simulink model "UAV_Fleet2"  (R2013b)
settings: Solver=ode1  StartTime=0.0  StopTime=300  FixedStep=simPars.SampleTime  RelTol=1e-3
undefined symbols (not defined in the file or in its folder): AC_Fleet, DiscIntNeverNeededParam, Earth, Env, eul_0, m, s, simPars, WGS84
libraries: simulink x23, Actuator_Lib x5, aerolib6dofsys x4, aerolibasang x3, instrumentlib x2, aerolibconvert2 x2, aerolibtransform2 x2, etargetslib x1, aerolibutil x1, aerolibatmos2 x1, aerolibobsolete x1, aerolibgravity2 x1
(part 1 of 2)
settings Model: Creator=Paul Freeman  LastModifiedBy=descobar
settings DataIOCC: LimitDataPoints=off  SignalLoggingSaveFormat=ModelDataLogs  SaveOutput=off  SignalLogging=off
settings OptimizationCC: ExpressionDepthLimit=2147483647
settings DebuggingCC: FcnCallInpInsideContextMsg=UseLocalSettings  StateNameClashWarn=warning
settings HardwareCC: ProdLargestAtomicInteger=Long  ProdLargestAtomicFloat=Double  ProdIntDivRoundTo=Zero  ProdEndianess=BigEndian  ProdHWDeviceType=Freescale->32-bit PowerPC
settings SFSimCC: SimParseCustomCode=off
settings GRTTargetCC: CombineOutputUpdateFcns=off  GRTInterface=on

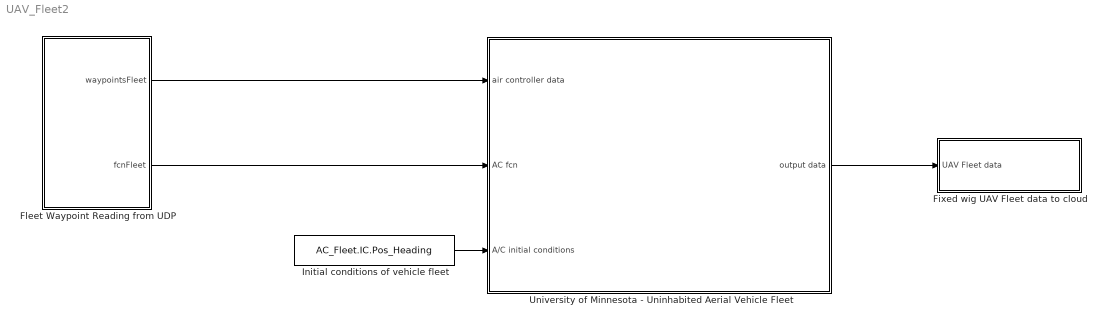
== system UAV_Fleet2 ==
  Fixed wig UAV Fleet data to cloud : Subsystem
  Fleet Waypoint Reading from UDP : Subsystem
  Initial conditions of vehicle fleet : Constant  Value=AC_Fleet.IC.Pos_Heading  VectorParams1D=off
  University of Minnesota - Uninhabited Aerial Vehicle Fleet : Subsystem  TreatAsAtomicUnit=on  mask{AC=AC_Fleet.AC, Env=Env, SampleTime=simPars.SampleTime}
      mask prompts: AC "Aircraft properties"; Env "Environmental parameters"; SampleTime "Sample time (sec)"
  wires:
  Initial conditions of vehicle fleet/1 -> University of Minnesota - Uninhabited Aerial Vehicle Fleet/3(A/C initial conditions)
  University of Minnesota - Uninhabited Aerial Vehicle Fleet/1(output data) -> Fixed wig UAV Fleet data to cloud/1(UAV Fleet data)
  Fleet Waypoint Reading from UDP/1(waypointsFleet) -> University of Minnesota - Uninhabited Aerial Vehicle Fleet/1(air controller data)
  Fleet Waypoint Reading from UDP/2(fcnFleet) -> University of Minnesota - Uninhabited Aerial Vehicle Fleet/2(AC fcn)

== system UAV_Fleet2/Fixed wig UAV Fleet data to cloud ==
  UAV Fleet data : Inport
  Rate Transition : RateTransition  OutPortSampleTime=simPars.SampleTime*5
  UDP Send : instrumentlib/UDP Send  Host=localhost  Port=9090  LocalPort=9091  EnableBlockingMode=on  ByteOrder=BigEndian
  wires:
  Rate Transition/1 -> UDP Send/1
  UAV Fleet data/1 -> Rate Transition/1

== system UAV_Fleet2/Fleet Waypoint Reading from UDP ==
  Byte Unpack : etargetslib/Byte Unpack  dimensions={[3],[2],[30], [1]}  datatypes={'uint8', 'uint16', 'double','uint16'}  byteAlign=1
  "DataBase " : MATLAB Function  TreatAsAtomicUnit=on
  Demux1 : Demux  Outputs=2
  UDP Receive : instrumentlib/UDP Receive  Host=localhost  Port=9040  LocalPort=9040  DataSize="[249    1]"  EnableBlockingMode=off  Timeout=10  SampleTime=0.02  DataType=uint8  ByteOrder=BigEndian
  term0 : Terminator
  term1 : Terminator
  waypointsFleet : Outport
  fcnFleet : Outport  Port=2
  wires:
  "DataBase "/1(dataFleet) -> waypointsFleet/1
  Demux1/2 -> "DataBase "/2(functionID)
  UDP Receive/2 -> "DataBase "/4(status)
  Demux1/1 -> "DataBase "/1(uavID)
  Byte Unpack/3 -> "DataBase "/3(dataUAV)
  Byte Unpack/2 -> Demux1/1
  UDP Receive/1 -> Byte Unpack/1
  "DataBase "/2(fcnFleet) -> fcnFleet/1
  Byte Unpack/1 -> term0/1
  Byte Unpack/4 -> term1/1

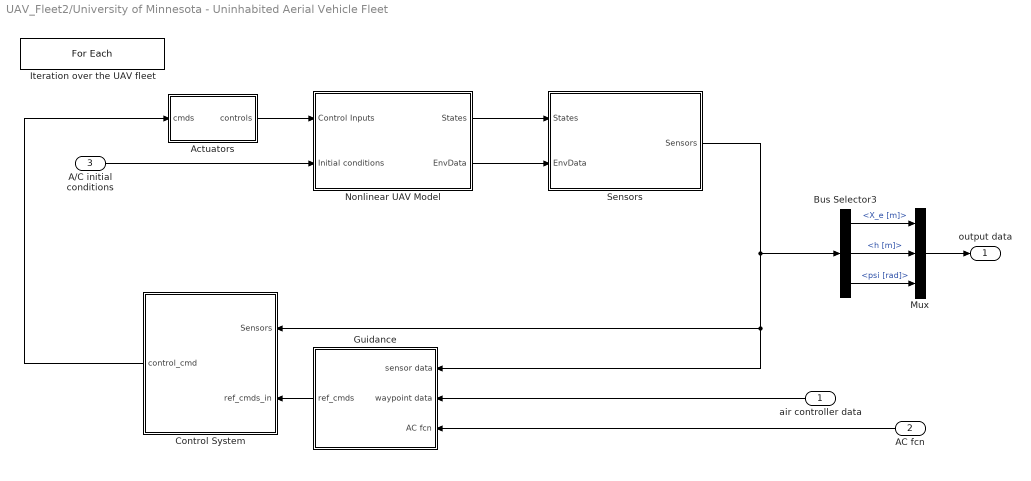
== system UAV_Fleet2/University of Minnesota - Uninhabited Aerial Vehicle Fleet ==
  air controller data : Inport  Partition=on  PartitionDimension=3  PartitionWidth=1
  AC fcn : Inport  Port=2  Partition=on  PartitionDimension=1  PartitionWidth=1
  A/C initial conditions : Inport  Port=3  Partition=on  PartitionDimension=2  PartitionWidth=1
  Actuators : Subsystem
  Bus Selector3 : BusSelector  OutputSignals=X_e [m],h [m],psi [rad]
  Control System : Subsystem  mask{control=AC.FC.control, IntegerTimeDelay=AC.FC.IntegerTimeDelay, TrimCondition=AC.TrimCondition, OperatingPoint=AC.OperatingPoint}
      mask prompts: control "Controller parameters"; IntegerTimeDelay "Integer Time Delay"; TrimCondition "Trim Condition"; OperatingPoint "Operating Point"
  "Guidance " : Subsystem
  Iteration over the UAV fleet : ForEach  DisableCoverage=on  IndexMode=One-based
  Mux : Mux  Inputs=3
  Nonlinear UAV Model : Subsystem  mask{TrimCondition=AC.TrimCondition}
      mask prompts: TrimCondition "Trim Condition"
  Sensors : Subsystem
  output data : Outport  ConcatenationDimension=1
  wires:
  Sensors/1(Sensors) -> "Guidance "/1(sensor data), Control System/1(Sensors), Bus Selector3/1
  Nonlinear UAV Model/1(States) -> Sensors/1(States)
  Nonlinear UAV Model/2(EnvData) -> Sensors/2(EnvData)
  Control System/1(control_cmd) -> Actuators/1(cmds)
  Actuators/1(controls) -> Nonlinear UAV Model/1(Control Inputs)
  "Guidance "/1(ref_cmds) -> Control System/2(ref_cmds_in)
  air controller data/1 -> "Guidance "/2(waypoint data)
  A/C initial conditions/1 -> Nonlinear UAV Model/2(Initial conditions)
  Bus Selector3/1 -> Mux/1  "<X_e [m]>"
  Bus Selector3/2 -> Mux/2  "<h [m]>"
  Mux/1 -> output data/1
  Bus Selector3/3 -> Mux/3  "<psi [rad]>"
  AC fcn/1 -> "Guidance "/3(AC fcn)

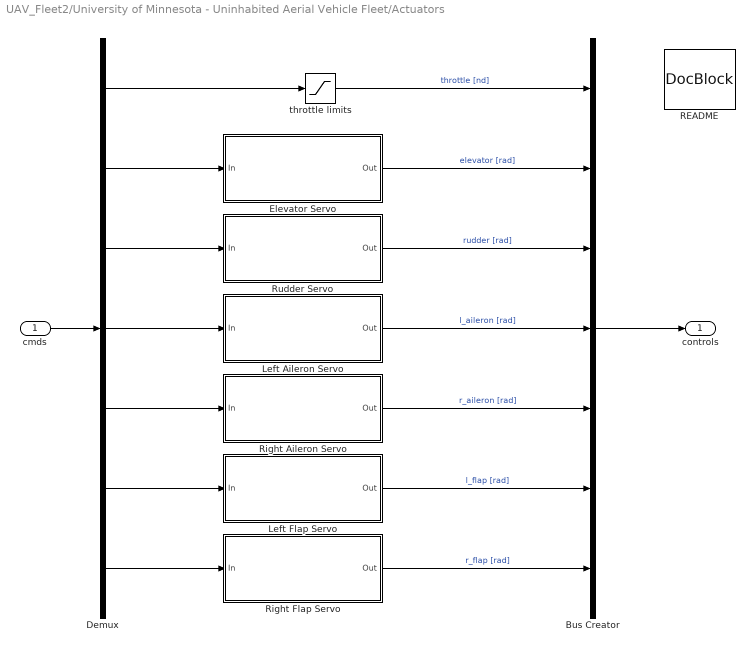
== system UAV_Fleet2/University of Minnesota - Uninhabited Aerial Vehicle Fleet/Actuators ==
  cmds : Inport
  Bus Creator : BusCreator  Inputs=7
  Demux : Demux  Outputs=7
  Elevator Servo : Subsystem  mask(Rate and Position Limited Servo){freq=AC.Actuator.elevator.BW, RL=AC.Actuator.elevator.RateLim, POS_hi=AC.Actuator.elevator.PosLim, POS_lo=AC.Actuator.elevator.NegLim}
      mask prompts: freq "Bandwidth, Hz"; RL "Rate Limit:"; POS_hi "Position Limit High:"; POS_lo "Position Limit Low:"
      mask help: First order transfer function: w/(s+w), with rate and position limits.
      mask Help:
      | This block models a first order servo with the initial condition
      | on the integrator set to the steady state value for constant input.
      | The servo is rate and position limited and those values are set
      | in the block parameters.
      mask Display:
      | text(.48,.55,sprintf('%3.1f Hz\nBW',freq),'horizontalAlignment','center');
      | 
      | text(0.18,0.45,sprintf('|d/dt|\n<%0.1f',RL),'horizontalAlignment','center');
      | 
      | text(0.88,0.85,num2str(POS_hi),'horizontalAlignment', 'center');
      | text(0.88,0.2,num2str(POS_lo),'horizontalAlignment', 'center');
      | text(0.73,0.5,'P\nL');
      | 
      | 
      | plot([0.83 0.87 0.93 0.97],[0.4 0.4 0.6 0.6]);
      | plot([0.81 0.99],[0.5 0.5]);
      | plot([0.9 0.9],[0.3 0.7]);
      | plot([0.81 0.99 0.99 0.81 0.81],[0.3 0.3 0.7 0.7 0.3]);
  Left Aileron Servo : Subsystem  mask(Rate and Position Limited Servo){freq=AC.Actuator.l_aileron.BW, RL=AC.Actuator.l_aileron.RateLim, POS_hi=AC.Actuator.l_aileron.PosLim, POS_lo=AC.Actuator.l_aileron.NegLim}
      mask prompts: freq "Bandwidth, Hz"; RL "Rate Limit:"; POS_hi "Position Limit High:"; POS_lo "Position Limit Low:"
      mask help: First order transfer function: w/(s+w), with rate and position limits.
      mask Help:
      | This block models a first order servo with the initial condition
      | on the integrator set to the steady state value for constant input.
      | The servo is rate and position limited and those values are set
      | in the block parameters.
      mask Display:
      | text(.48,.55,sprintf('%3.1f Hz\nBW',freq),'horizontalAlignment','center');
      | 
      | text(0.18,0.45,sprintf('|d/dt|\n<%0.1f',RL),'horizontalAlignment','center');
      | 
      | text(0.88,0.85,num2str(POS_hi),'horizontalAlignment', 'center');
      | text(0.88,0.2,num2str(POS_lo),'horizontalAlignment', 'center');
      | text(0.73,0.5,'P\nL');
      | 
      | 
      | plot([0.83 0.87 0.93 0.97],[0.4 0.4 0.6 0.6]);
      | plot([0.81 0.99],[0.5 0.5]);
      | plot([0.9 0.9],[0.3 0.7]);
      | plot([0.81 0.99 0.99 0.81 0.81],[0.3 0.3 0.7 0.7 0.3]);
  Left Flap Servo : Subsystem  mask(Rate and Position Limited Servo){freq=AC.Actuator.l_flap.BW, RL=AC.Actuator.l_flap.RateLim, POS_hi=AC.Actuator.l_flap.PosLim, POS_lo=AC.Actuator.l_flap.NegLim}
      mask prompts: freq "Bandwidth, Hz"; RL "Rate Limit:"; POS_hi "Position Limit High:"; POS_lo "Position Limit Low:"
      mask help: First order transfer function: w/(s+w), with rate and position limits.
      mask Help:
      | This block models a first order servo with the initial condition
      | on the integrator set to the steady state value for constant input.
      | The servo is rate and position limited and those values are set
      | in the block parameters.
      mask Display:
      | text(.48,.55,sprintf('%3.1f Hz\nBW',freq),'horizontalAlignment','center');
      | 
      | text(0.18,0.45,sprintf('|d/dt|\n<%0.1f',RL),'horizontalAlignment','center');
      | 
      | text(0.88,0.85,num2str(POS_hi),'horizontalAlignment', 'center');
      | text(0.88,0.2,num2str(POS_lo),'horizontalAlignment', 'center');
      | text(0.73,0.5,'P\nL');
      | 
      | 
      | plot([0.83 0.87 0.93 0.97],[0.4 0.4 0.6 0.6]);
      | plot([0.81 0.99],[0.5 0.5]);
      | plot([0.9 0.9],[0.3 0.7]);
      | plot([0.81 0.99 0.99 0.81 0.81],[0.3 0.3 0.7 0.7 0.3]);
  README : simulink/Model-Wide Utilities/DocBlock  DocumentType=Text
      content=|
      | Actuators
      |
      | This block implements first order, rate and position limited actuator
      | models for the aileron, elevator, rudder and flap channels. The throttle
      | does not have a servo, but is position limited.
      |
      | Parameters for these models are contained in the aircraft configuration
      | data structure variable, "AC". Specfically,
      |
      | >> AC.Actuator
      |
      | ans =
      |
      |      elevator: [1x1 struct]
      |     l_aileron: [1x1 struct]
      |     r_aileron: [1x1 struct]
      |        rudder: [1x1 struct]
      |        l_flap: [1x1 struct]
      |        r_flap: [1x1 struct]
      |      throttle: [1x1 struct]
      |
      | Control Inputs Sign Convention
      | Elevator: +TED
      | Rudder: +TEL
      | Ailerons: +TED, da = (da_R-da_L)/2
      | Flaps: +TED
      | Throttle: always positive
  Right Aileron Servo : Subsystem  mask(Rate and Position Limited Servo){freq=AC.Actuator.r_aileron.BW, RL=AC.Actuator.r_aileron.RateLim, POS_hi=AC.Actuator.r_aileron.PosLim, POS_lo=AC.Actuator.r_aileron.NegLim}
      mask prompts: freq "Bandwidth, Hz"; RL "Rate Limit:"; POS_hi "Position Limit High:"; POS_lo "Position Limit Low:"
      mask help: First order transfer function: w/(s+w), with rate and position limits.
      mask Help:
      | This block models a first order servo with the initial condition
      | on the integrator set to the steady state value for constant input.
      | The servo is rate and position limited and those values are set
      | in the block parameters.
      mask Display:
      | text(.48,.55,sprintf('%3.1f Hz\nBW',freq),'horizontalAlignment','center');
      | 
      | text(0.18,0.45,sprintf('|d/dt|\n<%0.1f',RL),'horizontalAlignment','center');
      | 
      | text(0.88,0.85,num2str(POS_hi),'horizontalAlignment', 'center');
      | text(0.88,0.2,num2str(POS_lo),'horizontalAlignment', 'center');
      | text(0.73,0.5,'P\nL');
      | 
      | 
      | plot([0.83 0.87 0.93 0.97],[0.4 0.4 0.6 0.6]);
      | plot([0.81 0.99],[0.5 0.5]);
      | plot([0.9 0.9],[0.3 0.7]);
      | plot([0.81 0.99 0.99 0.81 0.81],[0.3 0.3 0.7 0.7 0.3]);
  Right Flap Servo : Subsystem  mask(Rate and Position Limited Servo){freq=AC.Actuator.l_flap.BW, RL=AC.Actuator.l_flap.RateLim, POS_hi=AC.Actuator.l_flap.PosLim, POS_lo=AC.Actuator.l_flap.NegLim}
      mask prompts: freq "Bandwidth, Hz"; RL "Rate Limit:"; POS_hi "Position Limit High:"; POS_lo "Position Limit Low:"
      mask help: First order transfer function: w/(s+w), with rate and position limits.
      mask Help:
      | This block models a first order servo with the initial condition
      | on the integrator set to the steady state value for constant input.
      | The servo is rate and position limited and those values are set
      | in the block parameters.
      mask Display:
      | text(.48,.55,sprintf('%3.1f Hz\nBW',freq),'horizontalAlignment','center');
      | 
      | text(0.18,0.45,sprintf('|d/dt|\n<%0.1f',RL),'horizontalAlignment','center');
      | 
      | text(0.88,0.85,num2str(POS_hi),'horizontalAlignment', 'center');
      | text(0.88,0.2,num2str(POS_lo),'horizontalAlignment', 'center');
      | text(0.73,0.5,'P\nL');
      | 
      | 
      | plot([0.83 0.87 0.93 0.97],[0.4 0.4 0.6 0.6]);
      | plot([0.81 0.99],[0.5 0.5]);
      | plot([0.9 0.9],[0.3 0.7]);
      | plot([0.81 0.99 0.99 0.81 0.81],[0.3 0.3 0.7 0.7 0.3]);
  Rudder Servo : Subsystem  mask(Rate and Position Limited Servo){freq=AC.Actuator.rudder.BW, RL=AC.Actuator.rudder.RateLim, POS_hi=AC.Actuator.rudder.PosLim, POS_lo=AC.Actuator.rudder.NegLim}
      mask prompts: freq "Bandwidth, Hz"; RL "Rate Limit:"; POS_hi "Position Limit High:"; POS_lo "Position Limit Low:"
      mask help: First order transfer function: w/(s+w), with rate and position limits.
      mask Help:
      | This block models a first order servo with the initial condition
      | on the integrator set to the steady state value for constant input.
      | The servo is rate and position limited and those values are set
      | in the block parameters.
      mask Display:
      | text(.48,.55,sprintf('%3.1f Hz\nBW',freq),'horizontalAlignment','center');
      | 
      | text(0.18,0.45,sprintf('|d/dt|\n<%0.1f',RL),'horizontalAlignment','center');
      | 
      | text(0.88,0.85,num2str(POS_hi),'horizontalAlignment', 'center');
      | text(0.88,0.2,num2str(POS_lo),'horizontalAlignment', 'center');
      | text(0.73,0.5,'P\nL');
      | 
      | 
      | plot([0.83 0.87 0.93 0.97],[0.4 0.4 0.6 0.6]);
      | plot([0.81 0.99],[0.5 0.5]);
      | plot([0.9 0.9],[0.3 0.7]);
      | plot([0.81 0.99 0.99 0.81 0.81],[0.3 0.3 0.7 0.7 0.3]);
  throttle limits : Saturate  UpperLimit=AC.Actuator.throttle.PosLim  LowerLimit=AC.Actuator.throttle.NegLim
  controls : Outport
  wires:
  Bus Creator/1 -> controls/1
  cmds/1 -> Demux/1
  Demux/1 -> throttle limits/1
  throttle limits/1 -> Bus Creator/1  "throttle [nd]"
  Demux/2 -> Elevator Servo/1(In)
  Elevator Servo/1(Out) -> Bus Creator/2  "elevator [rad]"
  Demux/3 -> Rudder Servo/1(In)
  Rudder Servo/1(Out) -> Bus Creator/3  "rudder [rad]"
  Demux/4 -> Left Aileron Servo/1(In)
  Left Aileron Servo/1(Out) -> Bus Creator/4  "l_aileron [rad]"
  Demux/6 -> Left Flap Servo/1(In)
  Left Flap Servo/1(Out) -> Bus Creator/6  "l_flap [rad]"
  Right Aileron Servo/1(Out) -> Bus Creator/5  "r_aileron [rad]"
  Right Flap Servo/1(Out) -> Bus Creator/7  "r_flap [rad]"
  Demux/7 -> Right Flap Servo/1(In)
  Demux/5 -> Right Aileron Servo/1(In)

== system UAV_Fleet2/University of Minnesota - Uninhabited Aerial Vehicle Fleet/Control System ==
  note: See "Software\Documentation\UAV_controllaw_ICD.pdf" for
      | details on the input/output signals.
  Sensors : Inport
  ref_cmds_in : Inport  Port=2
  Bus Creator : BusCreator  Inputs=7
  Bus Selector1 : BusSelector  OutputSignals=phi [rad],theta [rad],psi [rad],p [rad/s],q [rad/s],r [rad/s],Ax [m/s^2],Ay [m/s^2],Az [m/s^2],h [m],V_s [m/s],alpha [rad],beta [rad],Geodetic Latitude [rad],Geodetic Longitude [rad],Altitude [m],Xdot [m/s],Ydot [m/s],Zdot [m/s]  OutputAsBus=on
  "Control_Algorithm " : Subsystem
  Demux : Demux  Outputs=7
  Integer Delay : Delay  DelayLength=IntegerTimeDelay  InitialCondition=repmat([TrimCondition.AttitudeIni;TrimCondition.RatesIni;TrimCondition.AccelsIni;OperatingPoint.op_report.Outputs(4).y;TrimCondition.WindAxesIni;TrimCondition.LLIni;0; zeros(3,1)],[1,IntegerTimeDelay])  InputProcessing=Inherited
  README : simulink/Model-Wide Utilities/DocBlock  DocumentType=Text
      content=|
      | Control Law Block
      |
      | This block uses Model Referencing to allow the user to easily switch out
      | control law implementations. An example usage would be first a user develops
      | a control law using simulink blocks. This controller is referred to as the
      | "simulink controller" and would be selected by setting the variable
      | "controller_mode" to 2. Once the development is completed, the user then
      | implements the Simulink controller into C-code suitable for integration
      | with the UAV software. This controller is referred to as the "flight code"
      | and would be selected by setting "controller_mode" to 1.
      |
      | This is done using the Simulink.Variant object. See the documentation for
      | more detail. The user can specify any number of variants for the Control
      | Software block; edit the ModelReferenceParameters by right-clicking this
      | block to set which Simulink model is reference for each Variant object.
      | Note that these objects must be present in the base workspace. It
      | is strongly recommended that you use the "simulink_controller.mdl" file as
      | a starting place and "Save As" to a different file name.
      |
      | In summary, to switch the Control Software, modify the "contoller_mode"
      | variable:
      | 1 = flight code controller (C implementation)
      | 2 = simulink controller (empty simulink model)
      |
      |
      | See "Software\Documentation\UAV_controllaw_ICD.pdf" for details on the
      | input/output signals.
      |
      | The control_cmd signal must have the following order:
      | throttle
      | elevator
      | rudder
      | l_aileron
      | r_aileron
      | l_flap
      | r_flap
      |
      | Control Inputs Sign Convention
      | TED = Trailing Edge Down
      | TEL = Trailing Edge Left
      | ------------------------
      | Elevator: +TED
      | Rudder: +TEL
      | Aileron: +TED, da = (da_R-da_L)/2
      | Throttle: always positive
      | Flap: +TED
      |
      |
      | The refrence command signal must have the following order:
      | 1. phi_cmd
      | 2. theta_cmd
      | 3. psi_cmd
      | 4. p_cmd
      | 5. q_cmd
      | 6. r_cmd
      | 7. V_s_cmd
      | 8. h_cmd
      | 9. gndtrk_cmd
      | 10. aoa_cmd
      | 11. aos_cmd
      | 12. gamma_cmd
      | Note the trimmed value of pitch angle theta is included in the reference
      | command. Use the Doublet Generator block (or other signal generating block)
      | to input reference commands to the Control Software.
  Terminator : Terminator
  "Trim setting " : Actuator_Lib/Trim setting 
  control_cmd : Outport
  wires:
  "Control_Algorithm "/1(control_cmd1) -> "Trim setting "/1
  Sensors/1 -> Bus Selector1/1
  ref_cmds_in/1 -> "Control_Algorithm "/2(ref_cmds)
  Bus Creator/1 -> control_cmd/1
  Demux/1 -> Bus Creator/1  "throttle [nd]"
  Demux/2 -> Bus Creator/2  "elevator [rad]"
  Demux/3 -> Bus Creator/3  "rudder [rad]"
  Demux/4 -> Bus Creator/4  "l_aileron [rad]"
  Demux/5 -> Bus Creator/5  "r_aileron [rad]"
  Demux/6 -> Bus Creator/6  "l_flap [rad]"
  Demux/7 -> Bus Creator/7  "r_flap [rad]"
  Integer Delay/1 -> "Control_Algorithm "/1(feedback)
  Bus Selector1/1 -> Integer Delay/1
  "Trim setting "/1 -> Demux/1
  "Control_Algorithm "/2(ref_cmds_out) -> Terminator/1

== system UAV_Fleet2/University of Minnesota - Uninhabited Aerial Vehicle Fleet/Guidance  ==
  note: See /Software/Documentation/UAV_controlaw_ICD.pdf
      | for details
  sensor data : Inport
  waypoint data : Inport  Port=2
  AC fcn : Inport  Port=3
  Bus Selector1 : BusSelector  OutputSignals=psi [rad]
  Bus Selector2 : BusSelector  OutputSignals=X_e [m].X [m],X_e [m].Y [m],X_e [m].Z [m]
  Constant : Constant  Value=0
  Ground track angle computation based on waypoints : MATLAB Function  TreatAsAtomicUnit=on
  Model Info : simulink/Model-Wide Utilities/Model Info  InitialBlockCM=None  Frame=on  DisplayStringWithTags=|  HorizontalTextAlignment=Center  LeftAlignmentValue=0.5  SourceBlockDiagram=UAV_Fleet2  TagMaxNumber=20
      | Ref Cmd Port Info
      | 
      | 1. phi_cmd
      | 2. theta_cmd
      | 3. psi_cmd
      | 4. p_cmd
      | 5. q_cmd
      | 6. r_cmd
      | 7. V_s_cmd
      | 8. h_cmd
      | 9. gndtrk_cmd
      | 10. aoa_cmd
      | 11. aos_cmd
      | 12. gamma_cmd
  Mux : Mux  Inputs=12
  Mux1 : Mux  Inputs=3
  ref_cmds : Outport
  wires:
  Mux/1 -> ref_cmds/1
  Bus Selector2/1 -> Mux1/1  "<X [m]>"
  Bus Selector2/2 -> Mux1/2  "<Y [m]>"
  Bus Selector2/3 -> Mux1/3  "<Z [m]>"
  sensor data/1 -> Bus Selector1/1, Bus Selector2/1
  Bus Selector1/1 -> Ground track angle computation based on waypoints/2(psi)  "<psi [rad]>"
  Mux1/1 -> Ground track angle computation based on waypoints/3(Pned)
  waypoint data/1 -> Ground track angle computation based on waypoints/1(waypoint)
  Ground track angle computation based on waypoints/2(psiTarget) -> Mux/9
  Constant/1 -> Mux/3, Mux/4, Mux/5, Mux/6, Mux/7, Mux/10, Mux/11, Mux/12, Mux/1, Mux/2
  Ground track angle computation based on waypoints/1(hCmd) -> Mux/8
  AC fcn/1 -> Ground track angle computation based on waypoints/4(fcn)

== system UAV_Fleet2/University of Minnesota - Uninhabited Aerial Vehicle Fleet/Nonlinear UAV Model ==
  Control Inputs : Inport
  Initial conditions : Inport  Port=2
  6DoF EOM : Subsystem  mask(6DoF EoM (Body Axis)){units=Metric (MKS), mtype=Fixed, rep=Euler Angles, xme_0=TrimCondition.InertialIni, Vm_0=TrimCondition.VelocitiesIni, pm_0=TrimCondition.RatesIni, mass_0=AC.Mass, mass_e=0.5, mass_f=2.0, inertia=AC.Inertia.Matrix, inertia_e=eye(3), inertia_f=2*eye(3), k_quat=1.0}
      mask prompts: mtype "Mass type:"; rep "Representation:"; xme_0 "Initial position in inertial axes [Xe,Ye,Ze]:"; Vm_0 "Initial velocity in body axes [U,v,w]:"; pm_0 "Initial body rotation rates [p,q,r]:"; mass_0 "Initial mass:"; mass_e "Empty mass:"; mass_f "Full mass:"; inertia_e "Empty inertia matrix:"; inertia_f "Full inertia matrix:"; k_quat "Gain for quaternion normalization:"
      mask help:
      | Integrate the six-degrees-of-freedom equations of motion in body axis.
      |
      | This block has been modified from the original Aerospace Blockset
      | implementation. The inertial position vector (Xe) is no longer computed.
      | The original block did not have a way to add steady state winds to the
      | inertial velocities (Ve) prior to integrating to get Xe. Therefore, this
      | step is performed in the Auxiliary Equations block.
      mask Help: eval('asbhelp(''sixdof_euler_angles'')');
      mask TypeOptions units: Metric (MKS) | English (Velocity in ft/s) | English (Velocity in kts)
      mask TypeOptions mtype: Fixed | Simple Variable | Custom Variable
      mask Callback mtype: aeroicon('aeroblk6dofbody');
      mask TypeOptions rep: Euler Angles | Quaternion
      mask Callback rep: aeroicon('aeroblk6dofbody');
  Auxiliary Equations : Subsystem
  Environment : Subsystem
  Forces and Moments : Subsystem
  Initial conditions1 : InportShadow  Port=2
  "Packaging initial Euler angles " : Subsystem
  README : simulink/Model-Wide Utilities/DocBlock  DocumentType=Text
      content=|
      | Nonlinear UAV Model
      |
      | This block implements the nonlinear UAV dynamics model. Beginning on the
      | left, the Forces and Moments block models all of the relevant external
      | forces and moments acting on the aircraft.
      |
      | The 6DoF EOM block implements the six degree of freedom, fixed mass,
      | flat, non-rotating Earth, rigid body equations of motion. This block has
      | been modified from the original Aerospace Blockset implementation. The
      | inertial position vector (Xe) is no longer computed. The original block
      | did not have a way to add steady state winds to the inertial velocities
      | (Ve) prior to integrating to get Xe. Therefore, this step is performed in
      | the Auxiliary Equations block.
      |
      | The Auxiliary Equations computes other relevant variables (such as angle
      | of attack, indicated airspeed, etc) from state data. In this block are
      | the Navigation equations.
      |
      | Finally, the Environment block has Aerospace Blockset models for Earth's
      | atmosphere, gravity, and magnetic fields. Winds are modeled in two
      | portions: steady and unsteady. The steady portion is defined by a speed
      | and direction, and is horizontal only. The unsteady portion is made up of
      | a wind shear model and a turbulence model.
  States : Outport
  EnvData : Outport  Port=2
  wires:
  6DoF EOM/6(Ab) -> Auxiliary Equations/6(A_b)
  6DoF EOM/5(pdot,qdot,rdot) -> Auxiliary Equations/5(AngAccel)
  6DoF EOM/4(p,q,r) -> Auxiliary Equations/4(AngVel)
  6DoF EOM/3(Vb) -> Auxiliary Equations/3(V_b)
  6DoF EOM/2(DCM) -> Auxiliary Equations/2(DCM)
  6DoF EOM/1(Euler) -> Auxiliary Equations/1(Euler)
  Control Inputs/1 -> Forces and Moments/1(Control Inputs)
  Forces and Moments/1(Total Force) -> 6DoF EOM/1(Forces)
  Forces and Moments/2(Total Moment) -> 6DoF EOM/2(Moments)
  Auxiliary Equations/1(States) -> States/1, Forces and Moments/2(States), Environment/1(States)
  Forces and Moments/3(nonGravForces) -> Auxiliary Equations/7(NonGravForces)
  Environment/1(EnvData) -> Forces and Moments/3(EnvData), Auxiliary Equations/8(EnvData), EnvData/1
  Initial conditions/1 -> Auxiliary Equations/9(Initial conditions)
  Initial conditions1/1 -> "Packaging initial Euler angles "/1(Position and heading)
  "Packaging initial Euler angles "/1(Initial Euler angles) -> 6DoF EOM/3(Euler ini. (rad))

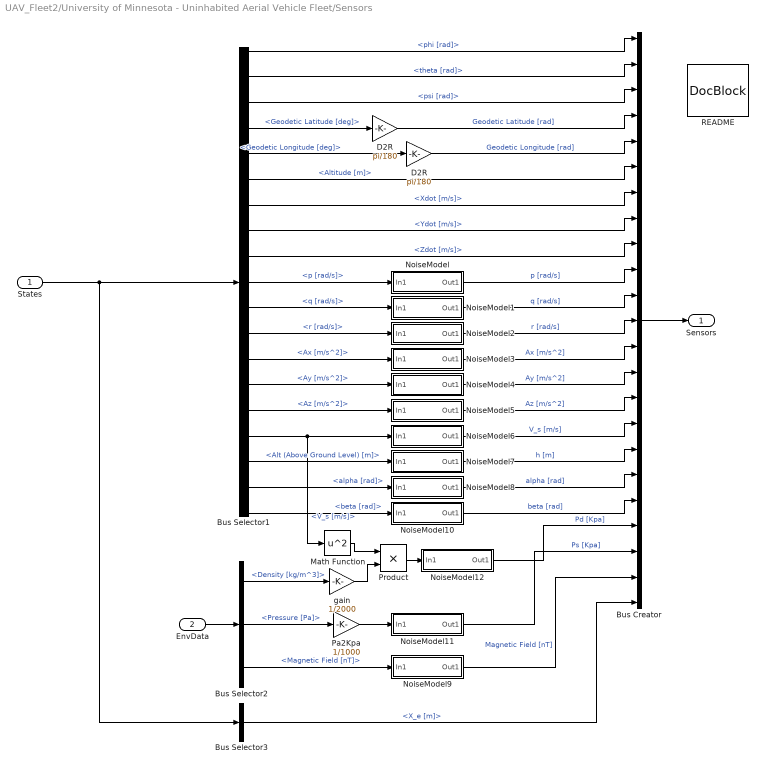
== system UAV_Fleet2/University of Minnesota - Uninhabited Aerial Vehicle Fleet/Sensors ==
  States : Inport
  EnvData : Inport  Port=2
  Bus Creator : BusCreator  Inputs=23
  Bus Selector1 : BusSelector  OutputSignals=Euler [rad].phi [rad],Euler [rad].theta [rad],Euler [rad].psi [rad],Nav.Geodetic Latitude [deg],Nav.Geodetic Longitude [deg],Nav.Altitude [m],V_e [m/s].Xdot [m/s],V_e [m/s].Ydot [m/s],V_e [m/s].Zdot [m/s],AngVel [rad/s].p [rad/s],AngVel [rad/s].q [rad/s],AngVel [rad/s].r [rad/s],Accels [m/s^2].Ax [m/s^2],Accels [m/s^2].Ay [m/s^2],Accels [m/s^2].Az [m/s^2],WindAxesParam.V_s [m/s],Nav.Alt (Above Ground Level) [m],WindAxesParam.alpha [rad],WindAxesParam.beta [rad]
  Bus Selector2 : BusSelector  OutputSignals=Density [kg/m^3],Pressure [Pa],Magnetic Field [nT]
  Bus Selector3 : BusSelector  OutputSignals=X_e [m]
  D2R : Gain  Gain=pi/180  SampleTime=SampleTime
  "D2R " : Gain  Gain=pi/180  SampleTime=SampleTime
  Math Function : Math  Operator=square  SaturateOnIntegerOverflow=on
  NoiseModel : Subsystem  mask(Sensor Model){noise_on=AC.Sensors.NoiseOn, sigma=AC.Sensors.IMU.p_noise, seed=878230, bias=AC.Sensors.IMU.p_bias, scf=AC.Sensors.IMU.p_scf, timestep=SampleTime}
      mask prompts: noise_on "on/off"; scf "scale factor:"
      mask help:
      | Add bias, scale factor, and white noise to a signal
      |
      | - 'on/off': 1 = noise on, 0 = noise off.
      | - 'sigma' : Standard deviation of white noise.
      | - 'seed'  : Random number seed.
      | - 'bias'  : Constant mean value offset of white noise.
      | - 'scale factor' : Scale factor applied to original signal.
      | - 'Timestep': Time step of the simulation
      mask Display: disp('bias/scf/noise')
  NoiseModel1 : Subsystem  mask(Sensor Model){noise_on=AC.Sensors.NoiseOn, sigma=AC.Sensors.IMU.q_noise, seed=878231, bias=AC.Sensors.IMU.q_bias, scf=AC.Sensors.IMU.q_scf, timestep=SampleTime}
      mask prompts: noise_on "on/off"; scf "scale factor:"
      mask help:
      | Add bias, scale factor, and white noise to a signal
      |
      | - 'on/off': 1 = noise on, 0 = noise off.
      | - 'sigma' : Standard deviation of white noise.
      | - 'seed'  : Random number seed.
      | - 'bias'  : Constant mean value offset of white noise.
      | - 'scale factor' : Scale factor applied to original signal.
      | - 'Timestep': Time step of the simulation
      mask Display: disp('bias/scf/noise')
  NoiseModel10 : Subsystem  mask(Sensor Model){noise_on=AC.Sensors.NoiseOn, sigma=AC.Sensors.AirData.beta_noise, seed=87828, bias=AC.Sensors.AirData.beta_bias, scf=AC.Sensors.AirData.beta_scf, timestep=SampleTime}
      mask prompts: noise_on "on/off"; scf "scale factor:"
      mask help:
      | Add bias, scale factor, and white noise to a signal
      |
      | - 'on/off': 1 = noise on, 0 = noise off.
      | - 'sigma' : Standard deviation of white noise.
      | - 'seed'  : Random number seed.
      | - 'bias'  : Constant mean value offset of white noise.
      | - 'scale factor' : Scale factor applied to original signal.
      | - 'Timestep': Time step of the simulation
      mask Display: disp('bias/scf/noise')
  NoiseModel11 : Subsystem  mask(Sensor Model){noise_on=AC.Sensors.NoiseOn, sigma=AC.Sensors.AirData.Ps_noise, seed=8782378, bias=AC.Sensors.AirData.Ps_bias, scf=AC.Sensors.AirData.Ps_scf, timestep=SampleTime}
      mask prompts: noise_on "on/off"; scf "scale factor:"
      mask help:
      | Add bias, scale factor, and white noise to a signal
      |
      | - 'on/off': 1 = noise on, 0 = noise off.
      | - 'sigma' : Standard deviation of white noise.
      | - 'seed'  : Random number seed.
      | - 'bias'  : Constant mean value offset of white noise.
      | - 'scale factor' : Scale factor applied to original signal.
      | - 'Timestep': Time step of the simulation
      mask Display: disp('bias/scf/noise')
  NoiseModel12 : Subsystem  mask(Sensor Model){noise_on=AC.Sensors.NoiseOn, sigma=AC.Sensors.AirData.Pd_noise, seed=87823, bias=AC.Sensors.AirData.Pd_bias, scf=AC.Sensors.AirData.Pd_scf, timestep=SampleTime}
      mask prompts: noise_on "on/off"; scf "scale factor:"
      mask help:
      | Add bias, scale factor, and white noise to a signal
      |
      | - 'on/off': 1 = noise on, 0 = noise off.
      | - 'sigma' : Standard deviation of white noise.
      | - 'seed'  : Random number seed.
      | - 'bias'  : Constant mean value offset of white noise.
      | - 'scale factor' : Scale factor applied to original signal.
      | - 'Timestep': Time step of the simulation
      mask Display: disp('bias/scf/noise')
  NoiseModel2 : Subsystem  mask(Sensor Model){noise_on=AC.Sensors.NoiseOn, sigma=AC.Sensors.IMU.r_noise, seed=878232, bias=AC.Sensors.IMU.r_bias, scf=AC.Sensors.IMU.r_scf, timestep=SampleTime}
      mask prompts: noise_on "on/off"; scf "scale factor:"
      mask help:
      | Add bias, scale factor, and white noise to a signal
      |
      | - 'on/off': 1 = noise on, 0 = noise off.
      | - 'sigma' : Standard deviation of white noise.
      | - 'seed'  : Random number seed.
      | - 'bias'  : Constant mean value offset of white noise.
      | - 'scale factor' : Scale factor applied to original signal.
      | - 'Timestep': Time step of the simulation
      mask Display: disp('bias/scf/noise')
  NoiseModel3 : Subsystem  mask(Sensor Model){noise_on=AC.Sensors.NoiseOn, sigma=AC.Sensors.IMU.ax_noise, seed=878233, bias=AC.Sensors.IMU.ax_bias, scf=AC.Sensors.IMU.ax_scf, timestep=SampleTime}
      mask prompts: noise_on "on/off"; scf "scale factor:"
      mask help:
      | Add bias, scale factor, and white noise to a signal
      |
      | - 'on/off': 1 = noise on, 0 = noise off.
      | - 'sigma' : Standard deviation of white noise.
      | - 'seed'  : Random number seed.
      | - 'bias'  : Constant mean value offset of white noise.
      | - 'scale factor' : Scale factor applied to original signal.
      | - 'Timestep': Time step of the simulation
      mask Display: disp('bias/scf/noise')
  NoiseModel4 : Subsystem  mask(Sensor Model){noise_on=AC.Sensors.NoiseOn, sigma=AC.Sensors.IMU.ay_noise, seed=878234, bias=AC.Sensors.IMU.ay_bias, scf=AC.Sensors.IMU.ay_scf, timestep=SampleTime}
      mask prompts: noise_on "on/off"; scf "scale factor:"
      mask help:
      | Add bias, scale factor, and white noise to a signal
      |
      | - 'on/off': 1 = noise on, 0 = noise off.
      | - 'sigma' : Standard deviation of white noise.
      | - 'seed'  : Random number seed.
      | - 'bias'  : Constant mean value offset of white noise.
      | - 'scale factor' : Scale factor applied to original signal.
      | - 'Timestep': Time step of the simulation
      mask Display: disp('bias/scf/noise')
  NoiseModel5 : Subsystem  mask(Sensor Model){noise_on=AC.Sensors.NoiseOn, sigma=AC.Sensors.IMU.az_noise, seed=878235, bias=AC.Sensors.IMU.az_bias, scf=AC.Sensors.IMU.az_scf, timestep=SampleTime}
      mask prompts: noise_on "on/off"; scf "scale factor:"
      mask help:
      | Add bias, scale factor, and white noise to a signal
      |
      | - 'on/off': 1 = noise on, 0 = noise off.
      | - 'sigma' : Standard deviation of white noise.
      | - 'seed'  : Random number seed.
      | - 'bias'  : Constant mean value offset of white noise.
      | - 'scale factor' : Scale factor applied to original signal.
      | - 'Timestep': Time step of the simulation
      mask Display: disp('bias/scf/noise')
  NoiseModel6 : Subsystem  mask(Sensor Model){noise_on=AC.Sensors.NoiseOn, sigma=AC.Sensors.AirData.ias_noise, seed=878236, bias=AC.Sensors.AirData.ias_bias, scf=AC.Sensors.AirData.ias_scf, timestep=SampleTime}
      mask prompts: noise_on "on/off"; scf "scale factor:"
      mask help:
      | Add bias, scale factor, and white noise to a signal
      |
      | - 'on/off': 1 = noise on, 0 = noise off.
      | - 'sigma' : Standard deviation of white noise.
      | - 'seed'  : Random number seed.
      | - 'bias'  : Constant mean value offset of white noise.
      | - 'scale factor' : Scale factor applied to original signal.
      | - 'Timestep': Time step of the simulation
      mask Display: disp('bias/scf/noise')
  NoiseModel7 : Subsystem  mask(Sensor Model){noise_on=AC.Sensors.NoiseOn, sigma=AC.Sensors.AirData.h_noise, seed=87828, bias=AC.Sensors.AirData.h_bias, scf=AC.Sensors.AirData.h_scf, timestep=SampleTime}
      mask prompts: noise_on "on/off"; scf "scale factor:"
      mask help:
      | Add bias, scale factor, and white noise to a signal
      |
      | - 'on/off': 1 = noise on, 0 = noise off.
      | - 'sigma' : Standard deviation of white noise.
      | - 'seed'  : Random number seed.
      | - 'bias'  : Constant mean value offset of white noise.
      | - 'scale factor' : Scale factor applied to original signal.
      | - 'Timestep': Time step of the simulation
      mask Display: disp('bias/scf/noise')
  NoiseModel8 : Subsystem  mask(Sensor Model){noise_on=AC.Sensors.NoiseOn, sigma=AC.Sensors.AirData.alpha_noise, seed=87828, bias=AC.Sensors.AirData.alpha_bias, scf=AC.Sensors.AirData.alpha_scf, timestep=SampleTime}
      mask prompts: noise_on "on/off"; scf "scale factor:"
      mask help:
      | Add bias, scale factor, and white noise to a signal
      |
      | - 'on/off': 1 = noise on, 0 = noise off.
      | - 'sigma' : Standard deviation of white noise.
      | - 'seed'  : Random number seed.
      | - 'bias'  : Constant mean value offset of white noise.
      | - 'scale factor' : Scale factor applied to original signal.
      | - 'Timestep': Time step of the simulation
      mask Display: disp('bias/scf/noise')
  NoiseModel9 : Subsystem  mask(Sensor Model){noise_on=AC.Sensors.NoiseOn, sigma=[AC.Sensors.IMU.hx_noise, AC.Sensors.IMU.hy_noise,AC.Sensors.IMU.hz_noise], seed=878237, bias=[AC.Sensors.IMU.hx_bias, AC.Sensors.IMU.hy_bias, AC.Sensors.IMU.hz_bias], scf=[AC.Sensors.IMU.hx_scf, AC.Sensors.IMU.hy_scf, AC.Sensors.IMU.hz_scf], timestep=SampleTime}
      mask prompts: noise_on "on/off"; scf "scale factor:"
      mask help:
      | Add bias, scale factor, and white noise to a signal
      |
      | - 'on/off': 1 = noise on, 0 = noise off.
      | - 'sigma' : Standard deviation of white noise.
      | - 'seed'  : Random number seed.
      | - 'bias'  : Constant mean value offset of white noise.
      | - 'scale factor' : Scale factor applied to original signal.
      | - 'Timestep': Time step of the simulation
      mask Display: disp('bias/scf/noise')
  Pa2Kpa : Gain  Gain=1/1000
  Product : Product  RndMeth=Zero
  README : simulink/Model-Wide Utilities/DocBlock  DocumentType=Text
      content=|
      | Sensors
      |
      | This block implements sensor models on selected signals. A generic block
      | is used that applies a bias, scale factor, and band limited white noise to
      | a given signal. The parameters for each block are stored in the aircraft
      | configuration data structure (AC):
      |
      | >> AC.Sensors
      |
      | ans =
      |
      |     NoiseOn: 1
      |         IMU: [1x1 struct]
      |     AirData: [1x1 struct]
      |
      | Note the "NoiseOn" boolean flag- by setting this flag to zero, the sensor
      | model will be disabled.
      |
      | Currently, the bias and scale factor errors are not used; only white noise
      | is applied.
  gain : Gain  Gain=1/2000
  Sensors : Outport
  wires:
  Bus Selector1/15 -> NoiseModel5/1(In1)  "<Az [m/s^2]>"
  Bus Selector1/14 -> NoiseModel4/1(In1)  "<Ay [m/s^2]>"
  Bus Selector1/13 -> NoiseModel3/1(In1)  "<Ax [m/s^2]>"
  Bus Selector1/12 -> NoiseModel2/1(In1)  "<r [rad/s]>"
  Bus Selector1/11 -> NoiseModel1/1(In1)  "<q [rad/s]>"
  Bus Selector1/10 -> NoiseModel/1(In1)  "<p [rad/s]>"
  States/1 -> Bus Selector3/1, Bus Selector1/1
  Bus Selector1/16 -> NoiseModel6/1(In1), Math Function/1  "<V_s [m/s]>"
  Bus Selector2/3 -> NoiseModel9/1(In1)  "<Magnetic Field [nT]>"
  Bus Selector1/17 -> NoiseModel7/1(In1)  "<Alt (Above Ground Level) [m]>"
  EnvData/1 -> Bus Selector2/1
  Bus Selector1/18 -> NoiseModel8/1(In1)  "<alpha [rad]>"
  Bus Selector1/19 -> NoiseModel10/1(In1)  "<beta [rad]>"
  Bus Selector2/2 -> Pa2Kpa/1  "<Pressure [Pa]>"
  Pa2Kpa/1 -> NoiseModel11/1(In1)
  Bus Selector2/1 -> gain/1  "<Density [kg/m^3]>"
  Math Function/1 -> Product/1
  gain/1 -> Product/2
  Product/1 -> NoiseModel12/1(In1)
  Bus Creator/1 -> Sensors/1
  Bus Selector1/1 -> Bus Creator/1  "<phi [rad]>"
  Bus Selector1/2 -> Bus Creator/2  "<theta [rad]>"
  Bus Selector1/3 -> Bus Creator/3  "<psi [rad]>"
  Bus Selector1/4 -> D2R/1  "<Geodetic Latitude [deg]>"
  Bus Selector1/5 -> "D2R "/1  "<Geodetic Longitude [deg]>"
  Bus Selector1/6 -> Bus Creator/6  "<Altitude [m]>"
  Bus Selector1/7 -> Bus Creator/7  "<Xdot [m/s]>"
  Bus Selector1/8 -> Bus Creator/8  "<Ydot [m/s]>"
  Bus Selector1/9 -> Bus Creator/9  "<Zdot [m/s]>"
  NoiseModel/1(Out1) -> Bus Creator/10  "p [rad/s]"
  NoiseModel1/1(Out1) -> Bus Creator/11  "q [rad/s]"
  NoiseModel2/1(Out1) -> Bus Creator/12  "r [rad/s]"
  NoiseModel3/1(Out1) -> Bus Creator/13  "Ax [m/s^2]"
  NoiseModel4/1(Out1) -> Bus Creator/14  "Ay [m/s^2]"
  NoiseModel5/1(Out1) -> Bus Creator/15  "Az [m/s^2]"
  NoiseModel6/1(Out1) -> Bus Creator/16  "V_s [m/s]"
  NoiseModel7/1(Out1) -> Bus Creator/17  "h [m]"
  NoiseModel8/1(Out1) -> Bus Creator/18  "alpha [rad]"
  NoiseModel10/1(Out1) -> Bus Creator/19  "beta [rad]"
  NoiseModel12/1(Out1) -> Bus Creator/20  "Pd [Kpa]"
  NoiseModel11/1(Out1) -> Bus Creator/21  "Ps [Kpa]"
  NoiseModel9/1(Out1) -> Bus Creator/22  "Magnetic Field [nT]"
  D2R/1 -> Bus Creator/4  "Geodetic Latitude [rad]"
  "D2R "/1 -> Bus Creator/5  "Geodetic Longitude [rad]"
  Bus Selector3/1 -> Bus Creator/23  "<X_e [m]>"

== system UAV_Fleet2/University of Minnesota - Uninhabited Aerial Vehicle Fleet/Actuators/Elevator Servo ==
  In : Inport
  Gain : Gain  Gain=2*pi*freq  SaturateOnIntegerOverflow=on  OutDataTypeStr=Inherit: Same as input  ParamDataTypeStr=Inherit: Same as input
  Integrator : Integrator  InitialConditionSource=external  LimitOutput=on  UpperSaturationLimit=POS_hi  LowerSaturationLimit=POS_lo  IgnoreLimit=on
  Rate Limiter : Saturate  UpperLimit=RL  LowerLimit=-RL
  Sum : Sum  Inputs=-+|  SaturateOnIntegerOverflow=on  InputSameDT=on  OutDataTypeStr=Inherit: Same as first input
  Out : Outport  PortDimensions=1
  wires:
  In/1 -> Sum/2, Integrator/2
  Rate Limiter/1 -> Integrator/1  "Ydot_lim"
  Integrator/1 -> Out/1, Sum/1  "Y"
  Sum/1 -> Gain/1  "Error"
  Gain/1 -> Rate Limiter/1  "Ydot"

== system UAV_Fleet2/University of Minnesota - Uninhabited Aerial Vehicle Fleet/Actuators/Left Aileron Servo ==
  In : Inport
  Gain : Gain  Gain=2*pi*freq  SaturateOnIntegerOverflow=on  OutDataTypeStr=Inherit: Same as input  ParamDataTypeStr=Inherit: Same as input
  Integrator : Integrator  InitialConditionSource=external  LimitOutput=on  UpperSaturationLimit=POS_hi  LowerSaturationLimit=POS_lo  IgnoreLimit=on
  Rate Limiter : Saturate  UpperLimit=RL  LowerLimit=-RL
  Sum : Sum  Inputs=-+|  SaturateOnIntegerOverflow=on  InputSameDT=on  OutDataTypeStr=Inherit: Same as first input
  Out : Outport  PortDimensions=1
  wires:
  In/1 -> Sum/2, Integrator/2
  Rate Limiter/1 -> Integrator/1  "Ydot_lim"
  Integrator/1 -> Out/1, Sum/1  "Y"
  Sum/1 -> Gain/1  "Error"
  Gain/1 -> Rate Limiter/1  "Ydot"

== system UAV_Fleet2/University of Minnesota - Uninhabited Aerial Vehicle Fleet/Actuators/Left Flap Servo ==
  In : Inport
  Gain : Gain  Gain=2*pi*freq  SaturateOnIntegerOverflow=on  OutDataTypeStr=Inherit: Same as input  ParamDataTypeStr=Inherit: Same as input
  Integrator : Integrator  InitialConditionSource=external  LimitOutput=on  UpperSaturationLimit=POS_hi  LowerSaturationLimit=POS_lo  IgnoreLimit=on
  Rate Limiter : Saturate  UpperLimit=RL  LowerLimit=-RL
  Sum : Sum  Inputs=-+|  SaturateOnIntegerOverflow=on  InputSameDT=on  OutDataTypeStr=Inherit: Same as first input
  Out : Outport  PortDimensions=1
  wires:
  In/1 -> Sum/2, Integrator/2
  Rate Limiter/1 -> Integrator/1  "Ydot_lim"
  Integrator/1 -> Out/1, Sum/1  "Y"
  Sum/1 -> Gain/1  "Error"
  Gain/1 -> Rate Limiter/1  "Ydot"

== system UAV_Fleet2/University of Minnesota - Uninhabited Aerial Vehicle Fleet/Actuators/Right Aileron Servo ==
  In : Inport
  Gain : Gain  Gain=2*pi*freq  SaturateOnIntegerOverflow=on  OutDataTypeStr=Inherit: Same as input  ParamDataTypeStr=Inherit: Same as input
  Integrator : Integrator  InitialConditionSource=external  LimitOutput=on  UpperSaturationLimit=POS_hi  LowerSaturationLimit=POS_lo  IgnoreLimit=on
  Rate Limiter : Saturate  UpperLimit=RL  LowerLimit=-RL
  Sum : Sum  Inputs=-+|  SaturateOnIntegerOverflow=on  InputSameDT=on  OutDataTypeStr=Inherit: Same as first input
  Out : Outport  PortDimensions=1
  wires:
  In/1 -> Sum/2, Integrator/2
  Rate Limiter/1 -> Integrator/1  "Ydot_lim"
  Integrator/1 -> Out/1, Sum/1  "Y"
  Sum/1 -> Gain/1  "Error"
  Gain/1 -> Rate Limiter/1  "Ydot"

== system UAV_Fleet2/University of Minnesota - Uninhabited Aerial Vehicle Fleet/Actuators/Right Flap Servo ==
  In : Inport
  Gain : Gain  Gain=2*pi*freq  SaturateOnIntegerOverflow=on  OutDataTypeStr=Inherit: Same as input  ParamDataTypeStr=Inherit: Same as input
  Integrator : Integrator  InitialConditionSource=external  LimitOutput=on  UpperSaturationLimit=POS_hi  LowerSaturationLimit=POS_lo  IgnoreLimit=on
  Rate Limiter : Saturate  UpperLimit=RL  LowerLimit=-RL
  Sum : Sum  Inputs=-+|  SaturateOnIntegerOverflow=on  InputSameDT=on  OutDataTypeStr=Inherit: Same as first input
  Out : Outport  PortDimensions=1
  wires:
  In/1 -> Sum/2, Integrator/2
  Rate Limiter/1 -> Integrator/1  "Ydot_lim"
  Integrator/1 -> Out/1, Sum/1  "Y"
  Sum/1 -> Gain/1  "Error"
  Gain/1 -> Rate Limiter/1  "Ydot"

== system UAV_Fleet2/University of Minnesota - Uninhabited Aerial Vehicle Fleet/Actuators/Rudder Servo ==
  In : Inport
  Gain : Gain  Gain=2*pi*freq  SaturateOnIntegerOverflow=on  OutDataTypeStr=Inherit: Same as input  ParamDataTypeStr=Inherit: Same as input
  Integrator : Integrator  InitialConditionSource=external  LimitOutput=on  UpperSaturationLimit=POS_hi  LowerSaturationLimit=POS_lo  IgnoreLimit=on
  Rate Limiter : Saturate  UpperLimit=RL  LowerLimit=-RL
  Sum : Sum  Inputs=-+|  SaturateOnIntegerOverflow=on  InputSameDT=on  OutDataTypeStr=Inherit: Same as first input
  Out : Outport  PortDimensions=1
  wires:
  In/1 -> Sum/2, Integrator/2
  Rate Limiter/1 -> Integrator/1  "Ydot_lim"
  Integrator/1 -> Out/1, Sum/1  "Y"
  Sum/1 -> Gain/1  "Error"
  Gain/1 -> Rate Limiter/1  "Ydot"

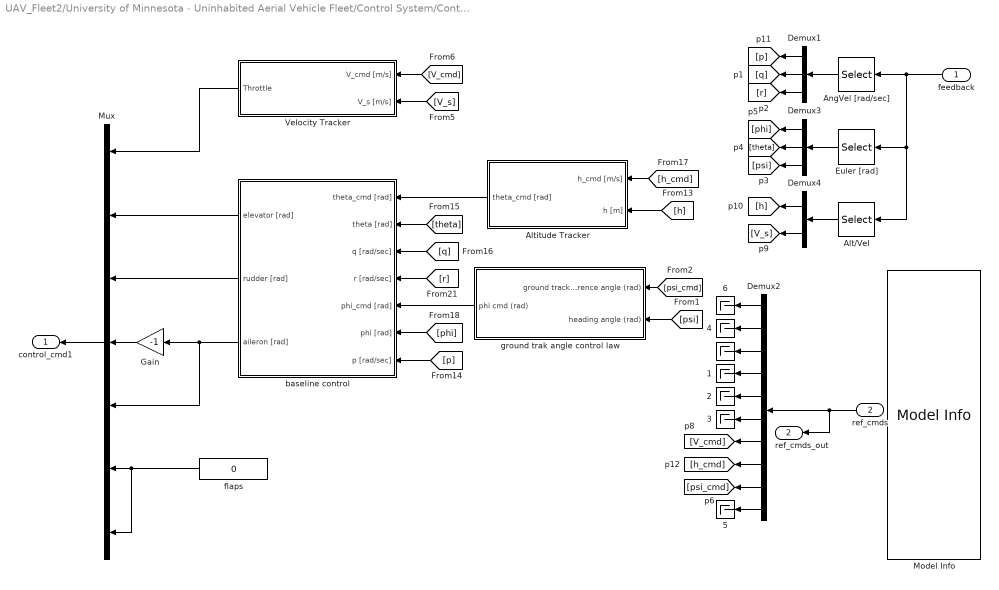
== system UAV_Fleet2/University of Minnesota - Uninhabited Aerial Vehicle Fleet/Control System/Control_Algorithm  ==
  feedback : Inport
  ref_cmds : Inport  Port=2
   {,1..6} (7 alike) : Terminator
  Alt/Vel : Selector  InputPortWidth=19  IndexOptions=Index vector (dialog)  Indices=[10:11]  OutputSizes=1
  Altitude Tracker : Subsystem
  AngVel [rad/sec] : Selector  InputPortWidth=19  IndexOptions=Index vector (dialog)  Indices=[4:6]  OutputSizes=1
  Demux1 : Demux  Outputs=3
  Demux2 : Demux  Outputs=[1 1 1 1 1 1 1 1 1 3]
  Demux3 : Demux  Outputs=3
  Demux4 : Demux  Outputs=2
  Euler [rad] : Selector  InputPortWidth=19  IndexOptions=Index vector (dialog)  Indices=[1:3]  OutputSizes=1
  Gain : Gain  Gain=-1
  Model Info : simulink/Model-Wide Utilities/Model Info  InitialBlockCM=None  Frame=on  DisplayStringWithTags=|  HorizontalTextAlignment=Center  LeftAlignmentValue=0.5  SourceBlockDiagram=UAV_Fleet2  TagMaxNumber=20
      | Ref Cmd Port Info
      | 
      | 1. phi_cmd
      | 2. theta_cmd
      | 3. psi_cmd
      | 4. p_cmd
      | 5. q_cmd
      | 6. r_cmd
      | 7. V_s_cmd
      | 8. h_cmd
      | 9. gndtrk_cmd
      | 10. aoa_cmd
      | 11. aos_cmd
      | 12. gamma_cmd
      | 13. signal_0
      | 14. signal_1
      | 15. signal_2
      | 16. signal_3
      | 17. signal_4
      | 18. signal_5
      | 19. signal_6
      | 20. signal_7
      | 21. signal_8
      | 22. signal_9
  Mux : Mux  Inputs=7
  Velocity Tracker : Subsystem
  baseline control : Subsystem  mask(Baseline Controller){pitch_gains=control.pitch_gains, roll_gains=control.roll_gains, yaw_damper_num=control.yaw_damper_num, yaw_damper_den=control.yaw_damper_den}
      mask prompts: pitch_gains "Pitch gains:"; roll_gains "Roll gains:"; yaw_damper_num "Yaw damper discrete transfer function numerator coefficients:"; yaw_damper_den "Yaw damper discrete transfer function denominator coefficients:"
      mask help:
      | The "Pitch gains" parameter takes a vector input in which the first term is the
      | proportional pitch tracking gain, the second term is the integral pitch
      | tracking gain, and the third term is the pitch rate proportional gain.
      |
      | The "Roll gains" parameter takes a vector input in which the first term is the
      | proportional roll tracking gain, the second term is the integral roll tracking
      | gain, and the third term is the roll rate proportional gain.
      |
      | The yaw damper parameters take vector inputs consisting of the discrete transfer
      | function numerator and denominator coefficients.
      |
      | See Mask help for a description of the control architecture.
      mask Help:
      | This is a simple baseline controller model for the Ultrastick UAVs.
      | For the pitch axis, there is a pitch damper consisting of a proportional
      | gain on the pitch rate. The output is subtracted from the output of a
      | PI control pitch angle tracker, and the result is sent to the elevator
      | command.
      | 
      | For the roll axis, there is a roll damper consisting of a proportional
      | gain (kp_RD) on the roll rate. The output is subtracted from the output of
      | a PI control roll angle tracker, and the result is sent to the aileron
      | command.
      | 
      | For the yaw axis, there is a discrete transfer function with input yawrate,
      | and output rudder.
  flaps : Constant  Value=0
  ground trak angle control law : Subsystem
  control_cmd1 : Outport
  ref_cmds_out : Outport  Port=2
  wires:
  flaps/1 -> Mux/6, Mux/7
  Mux/1 -> control_cmd1/1
  Demux3/1 -> [phi]
  feedback/1 -> AngVel [rad/sec]/1, Euler [rad]/1, Alt/Vel/1
  Demux4/1 -> [h]
  Demux4/2 -> [V_s]
  [theta] -> baseline control/2(theta [rad])
  Demux1/3 -> [r]
  Demux3/3 -> [psi]
  Gain/1 -> Mux/4
  Alt/Vel/1 -> Demux4/1
  Demux1/2 -> [q]
  Euler [rad]/1 -> Demux3/1
  AngVel [rad/sec]/1 -> Demux1/1
  Demux1/1 -> [p]
  Demux3/2 -> [theta]
  Demux2/5 -> " 2"/1
  Velocity Tracker/1("Throttle ") -> Mux/1
  Altitude Tracker/1(theta_cmd [rad]) -> baseline control/1(theta_cmd [rad])
  Demux2/6 -> " 3"/1
  Demux2/8 -> [h_cmd]
  [V_s] -> Velocity Tracker/2(V_s [m/s])
  ground trak angle control law/1(phi cmd (rad)) -> baseline control/5(phi_cmd [rad])
  [h] -> Altitude Tracker/2(h [m])
  baseline control/3(aileron [rad]) -> Gain/1, Mux/5
  baseline control/2(rudder [rad]) -> Mux/3
  baseline control/1(elevator [rad]) -> Mux/2
  ref_cmds/1 -> ref_cmds_out/1, Demux2/1
  Demux2/2 -> " 4"/1
  Demux2/9 -> [psi_cmd]
  [V_cmd] -> Velocity Tracker/1(V_cmd [m/s])
  [r] -> baseline control/4(r [rad/sec])
  [q] -> baseline control/3(q [rad/sec])
  Demux2/3 -> " "/1
  Demux2/4 -> " 1"/1
  Demux2/7 -> [V_cmd]
  [p] -> baseline control/7(p [rad/sec])
  [psi_cmd] -> ground trak angle control law/1(ground track reference angle (rad))
  Demux2/10 -> " 5"/1
  Demux2/1 -> " 6"/1
  [h_cmd] -> Altitude Tracker/1(h_cmd [m/s])
  [phi] -> baseline control/6(phi [rad])
  [psi] -> ground trak angle control law/2(heading angle (rad))

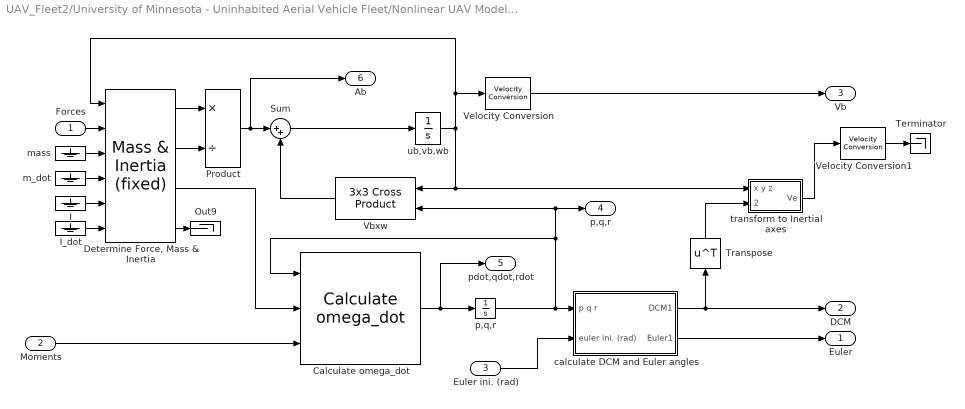
== system UAV_Fleet2/University of Minnesota - Uninhabited Aerial Vehicle Fleet/Nonlinear UAV Model/6DoF EOM ==
  Forces : Inport
  Moments : Inport  Port=2
  Euler ini. (rad) : Inport  Port=3
  Calculate omega_dot : aerolib6dofsys/Calculate omega_dot  SystemSampleTime=-1
  "Determine Force, Mass & Inertia" : aerolib6dofsys/Mass & Inertia (fixed)  SystemSampleTime=-1
  I : Ground
  I_dot : Ground
  Out9 : Terminator
  Product : Product  Inputs=*/  SaturateOnIntegerOverflow=on  OutDataTypeStr=Inherit: Same as first input
  Sum : Sum  Inputs=|++  SaturateOnIntegerOverflow=on
  Terminator : Terminator
  Transpose : Math  Operator=transpose  SaturateOnIntegerOverflow=on
  Vbxw : aerolibutil/3x3 Cross Product
  Velocity Conversion : aerolibconvert2/Velocity Conversion  IU=m/s  OU=m/s
  Velocity Conversion1 : aerolibconvert2/Velocity Conversion  IU=m/s  OU=m/s
  calculate DCM and Euler angles : Subsystem
  m_dot : Ground
  mass : Ground
  "p,q,r " : Integrator  InitialCondition=pm_0
  "transform to Inertial axes " : Subsystem  mask(Vector Transformation){}
      mask Display: disp('L_EB')
  ub,vb,wb : Integrator  InitialCondition=convvel(Vm_0,'m/s','m/s')
  Euler : Outport
  DCM : Outport  Port=2
  Vb : Outport  Port=3
  p,q,r : Outport  Port=4
  pdot,qdot,rdot : Outport  Port=5
  Ab : Outport  Port=6
  wires:
  Velocity Conversion1/1 -> Terminator/1
  Velocity Conversion/1 -> Vb/1
  "Determine Force, Mass & Inertia"/3 -> Calculate omega_dot/2
  calculate DCM and Euler angles/2(Euler1) -> Euler/1
  Vbxw/1 -> Sum/2
  ub,vb,wb/1 -> Velocity Conversion/1, "Determine Force, Mass & Inertia"/1, "transform to Inertial axes "/1(x y z), Vbxw/1
  Sum/1 -> ub,vb,wb/1
  "transform to Inertial axes "/1(Ve) -> Velocity Conversion1/1
  "p,q,r "/1 -> Calculate omega_dot/1, p,q,r/1, Vbxw/2, calculate DCM and Euler angles/1("p q r ")
  Moments/1 -> Calculate omega_dot/3
  Forces/1 -> "Determine Force, Mass & Inertia"/2
  Product/1 -> Sum/1, Ab/1
  calculate DCM and Euler angles/1(DCM1) -> Transpose/1, DCM/1
  Transpose/1 -> "transform to Inertial axes "/2(transform coefficients)
  mass/1 -> "Determine Force, Mass & Inertia"/3
  "Determine Force, Mass & Inertia"/2 -> Product/2
  m_dot/1 -> "Determine Force, Mass & Inertia"/4
  "Determine Force, Mass & Inertia"/4 -> Out9/1
  Calculate omega_dot/1 -> pdot,qdot,rdot/1, "p,q,r "/1
  I/1 -> "Determine Force, Mass & Inertia"/5
  I_dot/1 -> "Determine Force, Mass & Inertia"/6
  "Determine Force, Mass & Inertia"/1 -> Product/1
  Euler ini. (rad)/1 -> calculate DCM and Euler angles/2(euler ini. (rad))
